simulink model "tp2_EP"  (R2018b)
settings: Solver=VariableStepAuto  StartTime=0.0  StopTime=20  RelTol=1e-3
values from neighbouring files (symbols this model uses):
  A = R_t - R_inv    [TP1_ROB.m]    (also in Untitled.m = [0 1 0 0 ; 0 0 -9 0 ; 0 0 0 1;-1 0 0 0]; exocmee.m = [0 1 2/3;-1 -2 1;0 -3 1]; q1 (1).m = [0 1 0 0;0 0 -9 0;0 0 0 1;-1 0 0 0])
  F = 10    [ACMEE2.m]    (also in IDP3.m = @(s) (1/(1+1.4*s+s^2)); IDPDP.m = 6/((s+1).*(s+2).*(s+3)); TP2_DATA.m = [Y U]; precision_trap_simps.m = integral(g,x0,xn))
  J = 3/10-6./(t+1)+12./(2.*t+1)-6./(3.*t+1)+1./(2.*t)    [ACMEE2.m]    (also in simpson.m = h*(J1+2*J2+4*J3)/3)
  L = double(AP1)    [ACMEE1.m]    (also in TPACMEE1.m; Untitled.m = Kd'; exocmee.m = place(A',C',a2)'; simpson.m = (K1+2*K2+4*K3)*HX/3)
  P = 1/(C1*inv(-Abf)*B1)    [exocmee.m]
  R = ang2rot(alpha,beta,gamma)    [TP1_ROB.m]    (also in Untitled.m = 0.01; ang2rot.m = Rz * Ry * Rx; q1 (1).m = 1)
undefined symbols (not defined in the file or in its folder): Vf
settings Model: Creator=Abdou  LastModifiedBy=Abdou

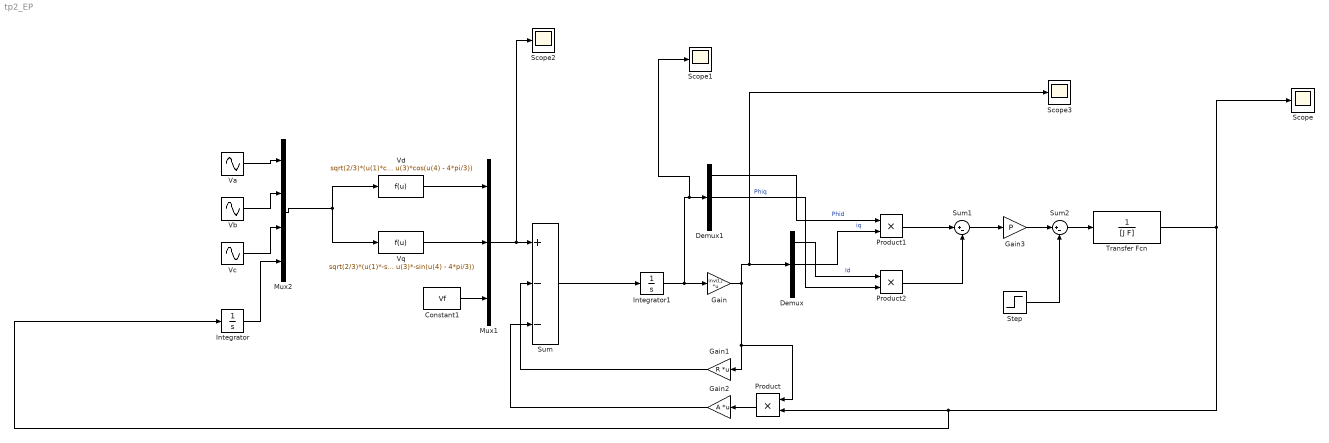
== system tp2_EP ==
  Constant1 : Constant  Value=Vf
  Demux : Demux  Outputs=3
  Demux1 : Demux  Outputs=3
  Gain : Gain  Gain=inv(L)  Multiplication=Matrix(K*u)
  Gain1 : Gain  Gain=R  Multiplication=Matrix(K*u)
  Gain2 : Gain  Gain=A  Multiplication=Matrix(K*u)
  Gain3 : Gain  Gain=P
  Integrator : Integrator
  Integrator1 : Integrator
  Mux1 : Mux  Inputs=3
  Mux2 : Mux
  Product : Product
  Product1 : Product
  Product2 : Product
  Scope{,1..3} (4 alike) : Scope
  Step : Step  After=20  SampleTime=0
  Sum : Sum  Inputs=+--
  Sum1 : Sum  Inputs=|+-
  Sum2 : Sum  Inputs=|+-
  Transfer Fcn : TransferFcn  Denominator=[J F]
  Va : Sin  Amplitude=220*sqrt(2)  Frequency=100*pi  SampleTime=0
  Vb : Sin  Amplitude=220*sqrt(2)  Frequency=100*pi  Phase=-2*pi/3  SampleTime=0
  Vc : Sin  Amplitude=220*sqrt(2)  Frequency=100*pi  Phase=-4*pi/3  SampleTime=0
  "Vd " : Fcn  Expr=sqrt(2/3)*(u(1)*cos(u(4)) + u(2)*cos(u(4)-2*pi/3) + u(3)*cos(u(4) - 4*pi/3))
  Vq : Fcn  Expr=sqrt(2/3)*(u(1)*-sin(u(4)) + u(2)*-sin(u(4)-2*pi/3) + u(3)*-sin(u(4) - 4*pi/3))
  wires:
  Transfer Fcn/1 -> Scope/1, Integrator/1, Product/2
  Mux1/1 -> Scope2/1, Sum/1
  Sum/1 -> Integrator1/1
  Integrator1/1 -> Scope1/1, Demux1/1, Gain/1
  Constant1/1 -> Mux1/3
  Gain/1 -> Scope3/1, Demux/1, Product/1, Gain1/1
  Product/1 -> Gain2/1
  Gain1/1 -> Sum/2
  Gain2/1 -> Sum/3
  Product1/1 -> Sum1/1
  Product2/1 -> Sum1/2
  Step/1 -> Sum2/2
  Sum1/1 -> Gain3/1
  Gain3/1 -> Sum2/1
  Sum2/1 -> Transfer Fcn/1
  Demux1/1 -> Product1/1  "Phid"
  Demux/2 -> Product1/2  "iq"
  Demux/1 -> Product2/1  "Id"
  Demux1/2 -> Product2/2  "Phiq"
  Va/1 -> Mux2/1
  Vb/1 -> Mux2/2
  Vc/1 -> Mux2/3
  Mux2/1 -> Vq/1, "Vd "/1
  "Vd "/1 -> Mux1/1
  Vq/1 -> Mux1/2
  Integrator/1 -> Mux2/4
